simulink model "Get_RE_RhythmCalc_Sig2Mbed_Tcontrol_paper_ver"  (R2013a)
settings: Solver=FixedStepDiscrete  StartTime=0.0  StopTime=65  RelTol=1e-3
values from neighbouring files (symbols this model uses):
  ts = 1/50    (= 0.02)    [arduino_setup.m]
libraries: arduino_io_lib x12, simulink x8
settings Model: Creator=cell  LastModifiedBy=cell
settings OptimizationCC: OptimizeModelRefInitCode=on  LifeSpan=1
settings DebuggingCC: CheckSSInitialOutputMsg=off  InheritedTsInSrcMsg=none  StrictBusMsg=Warning
settings HardwareCC: ProdBitPerInt=16  ProdBitPerPointer=8  ProdIntDivRoundTo=Zero  ProdEndianess=LittleEndian  ProdWordSize=8  ProdHWDeviceType=Atmel->AVR
settings RTWCC: SystemTargetFile=realtime.tlc  GenerateMakefile=off  TemplateMakefile=realtime.tmf  Description=Run on Target Hardware  RTWVerbose=off  ProcessScript=realtime_make_rtw_hook
settings CodeAppCC: IgnoreCustomStorageClasses=off
settings STFCustomTargetCC: TargetLibSuffix=.a  GenerateSampleERTMain=on  CombineOutputUpdateFcns=on  ERTCustomFileBanners=on  SupportContinuousTime=off  SupportNonInlinedSFcns=off  MATLABClassNameForMDSCustomization=Simulink.SoftwareTarget.ERTCustomization  SystemTargetFile=realtime.tlc
settings ERTTargetCC: ParMdlRefBuildCompliant=off  CompOptLevelCompliant=off  ConcurrentExecutionCompliant=off  ERTFirstTimeCompliant=off  ModelStepFunctionPrototypeControlCompliant=off  CPPClassGenCompliant=off  ERTCustomFileTemplate=realtime_file_process.tlc

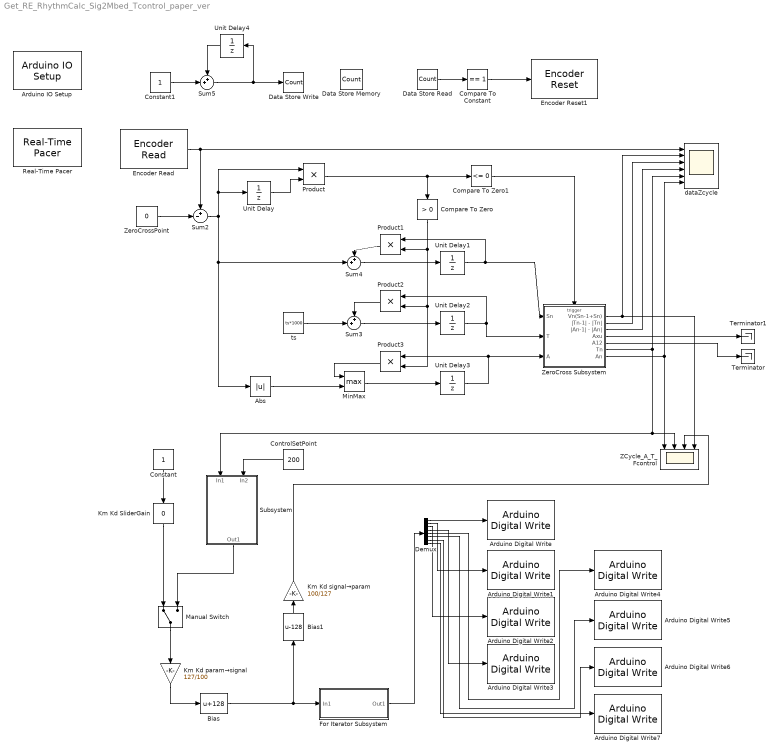
== system Get_RE_RhythmCalc_Sig2Mbed_Tcontrol_paper_ver ==
  Abs : Abs
  Arduino Digital Write : arduino_io_lib/Arduino Digital Write  arduinoVar=Existing workspace arduino variable #1  arduinoPin=6  T=ts
  Arduino Digital Write1 : arduino_io_lib/Arduino Digital Write  arduinoVar=Existing workspace arduino variable #1  arduinoPin=7  T=ts
  Arduino Digital Write2 : arduino_io_lib/Arduino Digital Write  arduinoVar=Existing workspace arduino variable #1  arduinoPin=8  T=ts
  Arduino Digital Write3 : arduino_io_lib/Arduino Digital Write  arduinoVar=Existing workspace arduino variable #1  arduinoPin=9  T=ts
  Arduino Digital Write4 : arduino_io_lib/Arduino Digital Write  arduinoVar=Existing workspace arduino variable #1  arduinoPin=10  T=ts
  Arduino Digital Write5 : arduino_io_lib/Arduino Digital Write  arduinoVar=Existing workspace arduino variable #1  arduinoPin=11  T=ts
  Arduino Digital Write6 : arduino_io_lib/Arduino Digital Write  arduinoVar=Existing workspace arduino variable #1  arduinoPin=12  T=ts
  Arduino Digital Write7 : arduino_io_lib/Arduino Digital Write  arduinoVar=Existing workspace arduino variable #1  arduinoPin=13  T=ts
  Arduino IO Setup : arduino_io_lib/Arduino IO Setup  Priority=3  arduinoVar=Existing workspace arduino variable #1  workspaceVarName=a  comPort=DEMO
  Bias : Bias  Bias=128
  Bias1 : Bias  Bias=-128
  Compare To Constant : simulink/Logic and Bit Operations/Compare To Constant  relop===  const=1  OutDataTypeStr=boolean
  Compare To Zero : simulink/Logic and Bit Operations/Compare To Zero  relop=>  OutDataTypeStr=boolean
  Compare To Zero1 : simulink/Logic and Bit Operations/Compare To Zero  relop=<=  OutDataTypeStr=boolean
  Constant : Constant
  Constant1 : Constant
  ControlSetPoint : Constant  Value=200
  Data Store Memory : DataStoreMemory  DataStoreName=Count  ReadBeforeWriteMsg=warning  WriteAfterWriteMsg=warning  WriteAfterReadMsg=warning
  Data Store Read : DataStoreRead  DataStoreName=Count
  Data Store Write : DataStoreWrite  DataStoreName=Count
  Demux : Demux  Outputs=8
  Encoder Read : arduino_io_lib/Encoder Read  arduinoVar=Existing workspace arduino variable #1  encNum=1  pinA=2  pinB=3  DbDl=0  T=ts
  Encoder Reset1 : arduino_io_lib/Encoder Reset  arduinoVar=Existing workspace arduino variable #1  encNum=1  T=ts
  For Iterator Subsystem : Subsystem  TreatAsAtomicUnit=on  mask{bits=8}
      mask prompts: bits "ビット数"
      mask Display: disp('Integer To Bit\nConvertor')
  Km Kd SliderGain : simulink/Math Operations/Slider Gain  low=-100  gain=0  high=100
  Km Kd param→signal : Gain  Gain=127/100
  Km Kd signal→param : Gain  Gain=100/127
  Manual Switch : ManualSwitch
  MinMax : MinMax  Function=max  Inputs=2  OutDataTypeStr=double
      settings: LockScale=on
  Product{,1..3} (4 alike) : Product
  Real-Time Pacer : arduino_io_lib/Real-Time Pacer  simTimePerRealTime=1
  Subsystem : Subsystem
  Sum2 : Sum  Inputs=+-|
  Sum3 : Sum  Inputs=++|
  Sum4 : Sum  Inputs=++|
  Sum5 : Sum  Inputs=++|
  Terminator : Terminator
  Terminator1 : Terminator
  Unit Delay{,1..4} (5 alike) : UnitDelay  SampleTime=-1
  ZCycle_A_T_Fcontrol : Scope  NumInputPorts=4
      settings: TimeRange=10  YMin=0~0~-50~-250  YMax=175~1400~50~250  SaveName=ZCycle_A_T_Fcontrol
  ZeroCross Subsystem : Subsystem  TreatAsAtomicUnit=on
  ZeroCrossPoint : Constant  Value=0
  dataZcycle : Scope  NumInputPorts=6
      settings: TimeRange=10  YMin=-250~-750~0~0~0~0  YMax=300~2500~400~225~700~500  SaveName=dataZcycle
  ts : Constant  Value=ts*1000
  wires:
  Encoder Read/1 -> dataZcycle/1, Sum2/1
  For Iterator Subsystem/1(Out1) -> Demux/1
  Demux/1 -> Arduino Digital Write/1
  Demux/2 -> Arduino Digital Write1/1
  Demux/3 -> Arduino Digital Write2/1
  Demux/4 -> Arduino Digital Write3/1
  Demux/5 -> Arduino Digital Write4/1
  Demux/6 -> Arduino Digital Write5/1
  Demux/7 -> Arduino Digital Write6/1
  Demux/8 -> Arduino Digital Write7/1
  ZeroCrossPoint/1 -> Sum2/2
  Compare To Zero1/1 -> ZeroCross Subsystem/Trigger
  Product/1 -> Compare To Zero1/1, Compare To Zero/1
  Sum2/1 -> Product/1, Unit Delay/1, Abs/1, Sum4/2
  Product2/1 -> Sum3/1
  Product1/1 -> Sum4/1
  Sum4/1 -> Unit Delay1/1
  ZeroCross Subsystem/3(|An-1| - |An|) -> dataZcycle/4
  Constant1/1 -> Sum5/2
  Sum5/1 -> Unit Delay4/1, Data Store Write/1
  ZeroCross Subsystem/2(|Tn-1| - |Tn|) -> dataZcycle/3
  Product3/1 -> MinMax/1
  Unit Delay4/1 -> Sum5/1
  Data Store Read/1 -> Compare To Constant/1
  Compare To Constant/1 -> Encoder Reset1/1
  ZeroCross Subsystem/6(Tn) -> dataZcycle/5, Subsystem/1(In1), ZCycle_A_T_Fcontrol/2
  ZeroCross Subsystem/7(An) -> dataZcycle/6, ZCycle_A_T_Fcontrol/1
  Constant/1 -> Km Kd SliderGain/1
  Bias/1 -> For Iterator Subsystem/1(In1), Bias1/1
  MinMax/1 -> Unit Delay3/1
  Unit Delay3/1 -> ZeroCross Subsystem/3(A), Product3/1
  Unit Delay2/1 -> ZeroCross Subsystem/2(T), Product2/1
  ts/1 -> Sum3/2
  Unit Delay1/1 -> ZeroCross Subsystem/1(Sn), Product1/1
  ZeroCross Subsystem/4(Axu) -> Terminator1/1
  ZeroCross Subsystem/5(A12) -> Terminator/1
  Subsystem/1(Out1) -> Manual Switch/2
  Unit Delay/1 -> Product/2
  Compare To Zero/1 -> Product3/2, Product2/2, Product1/2
  Sum3/1 -> Unit Delay2/1
  ZeroCross Subsystem/1(Vn(Sn-1+Sn)) -> ZCycle_A_T_Fcontrol/4, dataZcycle/2
  Abs/1 -> MinMax/2
  Manual Switch/1 -> Km Kd param→signal/1
  Km Kd param→signal/1 -> Bias/1
  Km Kd signal→param/1 -> ZCycle_A_T_Fcontrol/3
  Bias1/1 -> Km Kd signal→param/1
  ControlSetPoint/1 -> Subsystem/2(In2)
  Km Kd SliderGain/1 -> Manual Switch/1

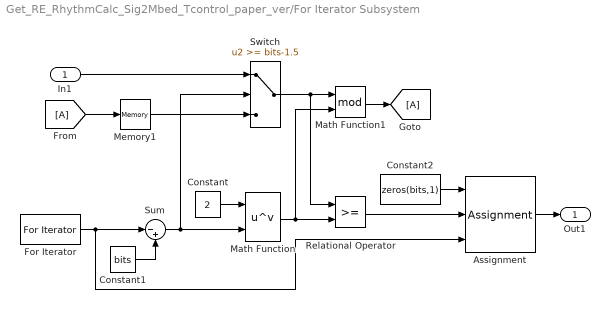
== system Get_RE_RhythmCalc_Sig2Mbed_Tcontrol_paper_ver/For Iterator Subsystem ==
  In1 : Inport
  Assignment : Assignment  IndexOptions=Index vector (port)  Indices=1  OutputSizes=[1 1]
  Constant : Constant  Value=2
  Constant1 : Constant  Value=bits
  Constant2 : Constant  Value=zeros(bits,1)  VectorParams1D=off
  For Iterator : ForIterator  IterationLimit=bits
  Math Function : Math  Operator=pow  SaturateOnIntegerOverflow=on
  Math Function1 : Math  Operator=mod  SaturateOnIntegerOverflow=on
  Memory1 : Memory  InheritSampleTime=on
  Relational Operator : RelationalOperator  OutDataTypeStr=float('double')
  Sum : Sum  Inputs=|-+
  Switch : Switch  Threshold=bits-1.5
  Out1 : Outport
  wires:
  For Iterator/1 -> Sum/1, Assignment/3
  Constant/1 -> Math Function/1
  Sum/1 -> Math Function/2, Switch/2
  Constant1/1 -> Sum/2
  Math Function/1 -> Math Function1/2, Relational Operator/2
  Switch/1 -> Math Function1/1, Relational Operator/1
  In1/1 -> Switch/1
  Memory1/1 -> Switch/3
  Assignment/1 -> Out1/1
  Constant2/1 -> Assignment/1
  Relational Operator/1 -> Assignment/2
  [A] -> Memory1/1
  Math Function1/1 -> [A]

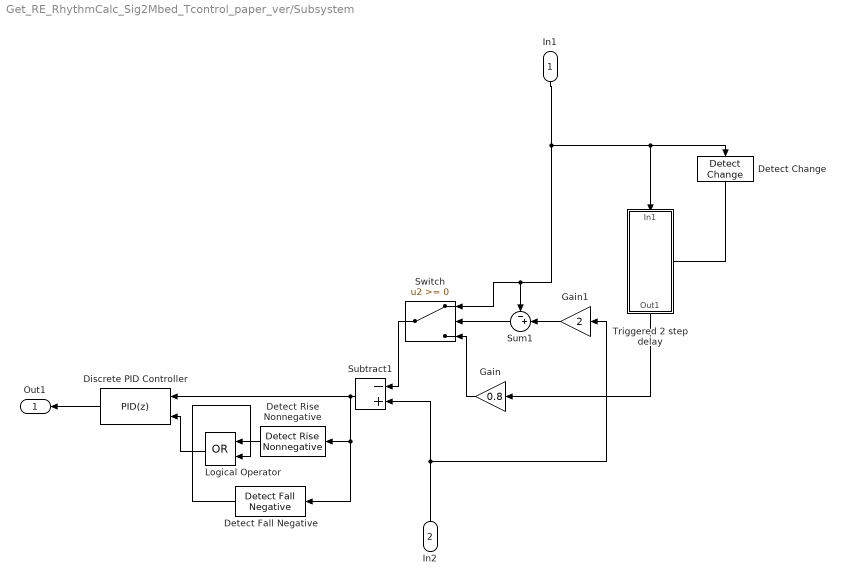
== system Get_RE_RhythmCalc_Sig2Mbed_Tcontrol_paper_ver/Subsystem ==
  In1 : Inport
  In2 : Inport  Port=2
  Detect Change : simulink/Logic and Bit Operations/Detect Change  vinit=0  InputProcessing=Inherited  OutDataTypeStr=boolean
  Detect Fall Negative : simulink/Logic and Bit Operations/Detect Fall Negative  vinit=0  InputProcessing=Inherited  OutDataTypeStr=boolean
  Detect Rise Nonnegative : simulink/Logic and Bit Operations/Detect Rise Nonnegative  vinit=0  InputProcessing=Inherited  OutDataTypeStr=boolean
  Discrete PID Controller : simulink/Continuous/PID Controller  Controller=PID  TimeDomain=Discrete-time  SampleTime=-1  IntegratorMethod=Forward Euler  FilterMethod=Forward Euler  Form=Parallel  P=0.2  I=0.05  D=0  N=100  InitialConditionSource=internal  InitialConditionForIntegrator=0  InitialConditionForFilter=0  ExternalReset=rising  LimitOutput=on  UpperSaturationLimit=50  LowerSaturationLimit=-50  LinearizeAsGain=off  AntiWindupMode=none  Kb=1  TrackingMode=off  Kt=1  PParamMin=[]  PParamMax=[]  IParamMin=[]  IParamMax=[]  DParamMin=[]  DParamMax=[]  NParamMin=[]  NParamMax=[]  KbParamMin=[]  KbParamMax=[]  KtParamMin=[]  KtParamMax=[]  POutMin=[]  POutMax=[]  IOutMin=[]  IOutMax=[]  DOutMin=[]  DOutMax=[]  NOutMin=[]  NOutMax=[]  KbOutMin=[]  KbOutMax=[]  KtOutMin=[]  KtOutMax=[]  IntegratorOutMin=[]  IntegratorOutMax=[]  FilterOutMin=[]  FilterOutMax=[]  SumOutMin=[]  SumOutMax=[]  SumI1OutMin=[]  SumI1OutMax=[]  SumI2OutMin=[]  SumI2OutMax=[]  SumI3OutMin=[]  SumI3OutMax=[]  SumDOutMin=[]  SumDOutMax=[]  SaturationOutMin=[]  SaturationOutMax=[]  IntegratorContinuousStateAttributes=''  IntegratorStateMustResolveToSignalObject=off  IntegratorRTWStateStorageClass=Auto  FilterContinuousStateAttributes=''  FilterStateMustResolveToSignalObject=off  FilterRTWStateStorageClass=Auto
  Gain : Gain  Gain=0.8
  Gain1 : Gain  Gain=2
  Logical Operator : Logic  Operator=OR  AllPortsSameDT=off  OutDataTypeStr=boolean
  Subtract1 : Sum  Inputs=-+
  Sum1 : Sum  Inputs=-+|
  Switch : Switch
  Triggered 2 step delay : Subsystem  TreatAsAtomicUnit=on
  Out1 : Outport
  wires:
  In1/1 -> Sum1/1, Switch/1, Detect Change/1, Triggered 2 step delay/1(In1)
  In2/1 -> Gain1/1, Subtract1/2
  Subtract1/1 -> Detect Fall Negative/1, Detect Rise Nonnegative/1, Discrete PID Controller/1
  Switch/1 -> Subtract1/1
  Gain/1 -> Switch/3
  Gain1/1 -> Sum1/2
  Detect Change/1 -> Triggered 2 step delay/Trigger
  Triggered 2 step delay/1(Out1) -> Gain/1
  Sum1/1 -> Switch/2
  Logical Operator/1 -> Discrete PID Controller/2
  Detect Rise Nonnegative/1 -> Logical Operator/1
  Detect Fall Negative/1 -> Logical Operator/2
  Discrete PID Controller/1 -> Out1/1

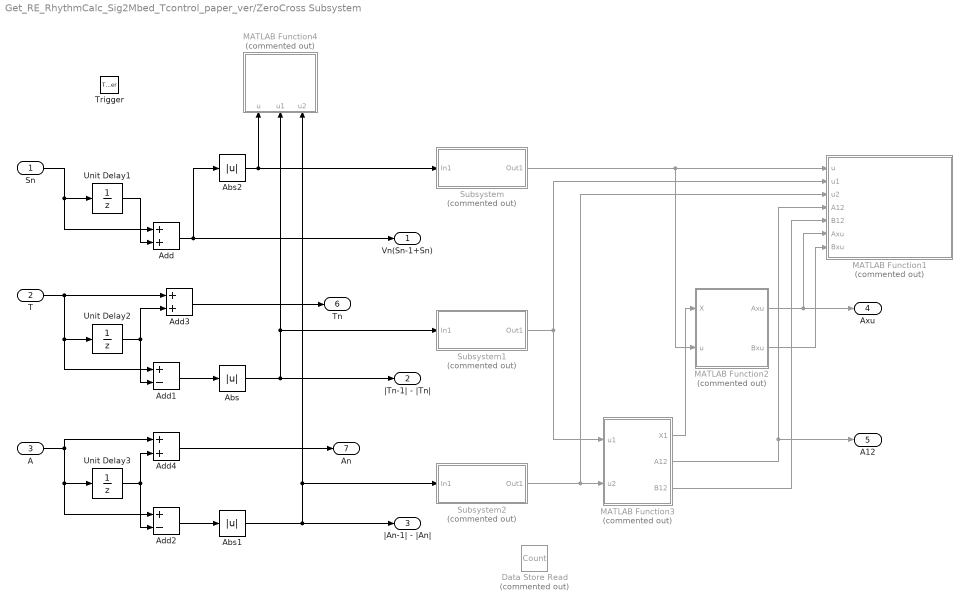
== system Get_RE_RhythmCalc_Sig2Mbed_Tcontrol_paper_ver/ZeroCross Subsystem ==
  Sn : Inport
  T : Inport  Port=2
  A : Inport  Port=3
  Trigger : TriggerPort
  Abs : Abs
  Abs1 : Abs
  Abs2 : Abs
  Add : Sum
  Add1 : Sum  Inputs=+-
  Add2 : Sum  Inputs=+-
  Add3 : Sum
  Add4 : Sum
  Data Store Read : DataStoreRead  Commented=on  DataStoreName=Count
  MATLAB Function1 : MATLAB Function  Commented=on  TreatAsAtomicUnit=on
  MATLAB Function2 : MATLAB Function  Commented=on  TreatAsAtomicUnit=on
  MATLAB Function3 : MATLAB Function  Commented=on  TreatAsAtomicUnit=on
  MATLAB Function4 : MATLAB Function  Commented=on  TreatAsAtomicUnit=on
  Subsystem : Subsystem  Commented=on
  Subsystem1 : Subsystem  Commented=on
  Subsystem2 : Subsystem  Commented=on
  Unit Delay1 : UnitDelay  SampleTime=-1
  Unit Delay2 : UnitDelay  SampleTime=-1
  Unit Delay3 : UnitDelay  SampleTime=-1
  Vn(Sn-1+Sn) : Outport
  |Tn-1| - |Tn| : Outport  Port=2
  |An-1| - |An| : Outport  Port=3
  Axu : Outport  Port=4
  A12 : Outport  Port=5
  Tn : Outport  Port=6
  An : Outport  Port=7
  wires:
  Unit Delay1/1 -> Add/2
  Sn/1 -> Add/1, Unit Delay1/1
  Unit Delay2/1 -> Add1/2, Add3/2
  T/1 -> Add1/1, Unit Delay2/1, Add3/1
  Add1/1 -> Abs/1
  Unit Delay3/1 -> Add4/2, Add2/2
  Add2/1 -> Abs1/1
  Abs1/1 -> |An-1| - |An|/1, MATLAB Function4/3(u2), Subsystem2/1(In1)
  Add/1 -> Abs2/1, Vn(Sn-1+Sn)/1
  Abs/1 -> |Tn-1| - |Tn|/1, Subsystem1/1(In1), MATLAB Function4/2(u1)
  Abs2/1 -> Subsystem/1(In1), MATLAB Function4/1(u)
  Subsystem1/1(Out1) -> MATLAB Function1/2(u1), MATLAB Function3/1(u1)
  Subsystem2/1(Out1) -> MATLAB Function1/3(u2), MATLAB Function3/2(u2)
  MATLAB Function3/1(X1) -> MATLAB Function2/1(X)
  Subsystem/1(Out1) -> MATLAB Function1/1(u), MATLAB Function2/2(u)
  MATLAB Function2/1(Axu) -> Axu/1, MATLAB Function1/6(Axu)
  MATLAB Function2/2(Bxu) -> MATLAB Function1/7(Bxu)
  MATLAB Function3/3(B12) -> MATLAB Function1/5(B12)
  MATLAB Function3/2(A12) -> MATLAB Function1/4(A12), A12/1
  Add3/1 -> Tn/1
  A/1 -> Unit Delay3/1, Add2/1, Add4/1
  Add4/1 -> An/1

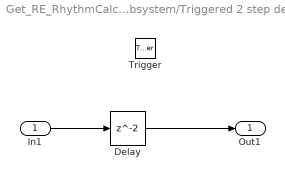
== system Get_RE_RhythmCalc_Sig2Mbed_Tcontrol_paper_ver/Subsystem/Triggered 2 step delay ==
  In1 : Inport
  Trigger : TriggerPort
  Delay : Delay
  Out1 : Outport
  wires:
  In1/1 -> Delay/1
  Delay/1 -> Out1/1

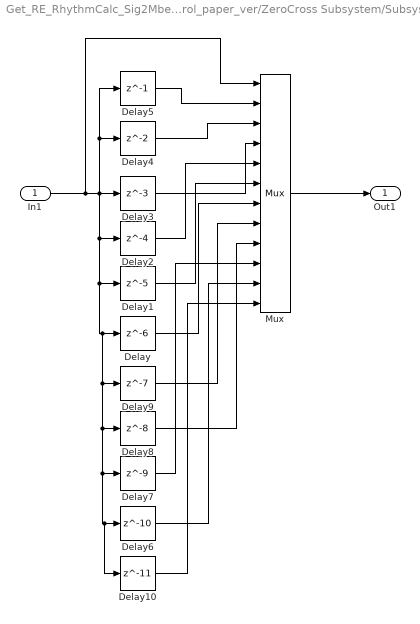
== system Get_RE_RhythmCalc_Sig2Mbed_Tcontrol_paper_ver/ZeroCross Subsystem/Subsystem ==
  In1 : Inport
  Delay : Delay  DelayLength=6
  Delay1 : Delay  DelayLength=5
  Delay10 : Delay  DelayLength=11
  Delay2 : Delay  DelayLength=4
  Delay3 : Delay  DelayLength=3
  Delay4 : Delay
  Delay5 : Delay  DelayLength=1
  Delay6 : Delay  DelayLength=10
  Delay7 : Delay  DelayLength=9
  Delay8 : Delay  DelayLength=8
  Delay9 : Delay  DelayLength=7
  Mux : Mux  Inputs=12
  Out1 : Outport
  wires:
  In1/1 -> Delay5/1, Delay4/1, Delay10/1, Delay6/1, Delay7/1, Delay8/1, Delay9/1, Delay/1, Delay1/1, Delay2/1, Delay3/1, Mux/1
  Delay5/1 -> Mux/2
  Delay4/1 -> Mux/3
  Delay3/1 -> Mux/4
  Delay2/1 -> Mux/5
  Delay1/1 -> Mux/6
  Delay/1 -> Mux/7
  Mux/1 -> Out1/1
  Delay9/1 -> Mux/8
  Delay8/1 -> Mux/9
  Delay7/1 -> Mux/10
  Delay6/1 -> Mux/11
  Delay10/1 -> Mux/12

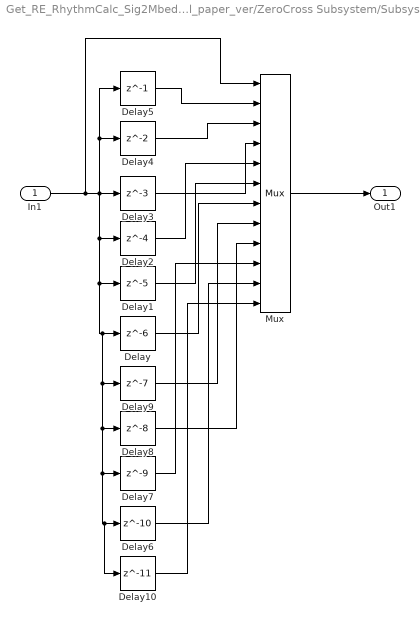
== system Get_RE_RhythmCalc_Sig2Mbed_Tcontrol_paper_ver/ZeroCross Subsystem/Subsystem1 ==
  In1 : Inport
  Delay : Delay  DelayLength=6
  Delay1 : Delay  DelayLength=5
  Delay10 : Delay  DelayLength=11
  Delay2 : Delay  DelayLength=4
  Delay3 : Delay  DelayLength=3
  Delay4 : Delay
  Delay5 : Delay  DelayLength=1
  Delay6 : Delay  DelayLength=10
  Delay7 : Delay  DelayLength=9
  Delay8 : Delay  DelayLength=8
  Delay9 : Delay  DelayLength=7
  Mux : Mux  Inputs=12
  Out1 : Outport
  wires:
  Delay10/1 -> Mux/12
  Delay6/1 -> Mux/11
  Delay7/1 -> Mux/10
  Delay8/1 -> Mux/9
  Delay9/1 -> Mux/8
  Mux/1 -> Out1/1
  Delay/1 -> Mux/7
  Delay1/1 -> Mux/6
  Delay2/1 -> Mux/5
  Delay3/1 -> Mux/4
  Delay4/1 -> Mux/3
  Delay5/1 -> Mux/2
  In1/1 -> Mux/1, Delay3/1, Delay2/1, Delay1/1, Delay/1, Delay9/1, Delay8/1, Delay7/1, Delay6/1, Delay10/1, Delay4/1, Delay5/1

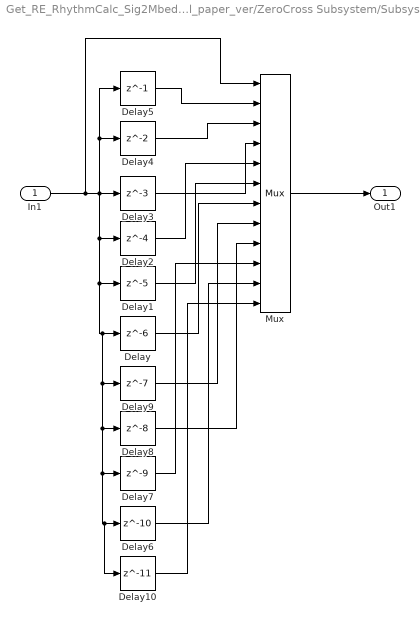
== system Get_RE_RhythmCalc_Sig2Mbed_Tcontrol_paper_ver/ZeroCross Subsystem/Subsystem2 ==
  In1 : Inport
  Delay : Delay  DelayLength=6
  Delay1 : Delay  DelayLength=5
  Delay10 : Delay  DelayLength=11
  Delay2 : Delay  DelayLength=4
  Delay3 : Delay  DelayLength=3
  Delay4 : Delay
  Delay5 : Delay  DelayLength=1
  Delay6 : Delay  DelayLength=10
  Delay7 : Delay  DelayLength=9
  Delay8 : Delay  DelayLength=8
  Delay9 : Delay  DelayLength=7
  Mux : Mux  Inputs=12
  Out1 : Outport
  wires:
  In1/1 -> Delay5/1, Delay4/1, Delay10/1, Delay6/1, Delay7/1, Delay8/1, Delay9/1, Delay/1, Delay1/1, Delay2/1, Delay3/1, Mux/1
  Delay5/1 -> Mux/2
  Delay4/1 -> Mux/3
  Delay3/1 -> Mux/4
  Delay2/1 -> Mux/5
  Delay1/1 -> Mux/6
  Delay/1 -> Mux/7
  Mux/1 -> Out1/1
  Delay9/1 -> Mux/8
  Delay8/1 -> Mux/9
  Delay7/1 -> Mux/10
  Delay6/1 -> Mux/11
  Delay10/1 -> Mux/12

== matlab function Get_RE_RhythmCalc_Sig2Mbed_Tcontrol_paper_ver/ZeroCross Subsystem/MATLAB Function2 ==
  data: X input; u input; Axu output; Bxu output
function [ Axu , Bxu]  = ols_method2( X, u )
%#codegen

% coder.extrinsic('polyfit')
    
% if length(u1) == 7
%     [au12 , bu12]= polyfit(u1 , u2 , 1);
% end

% if Count ==1
%     Sx = sum(u1(1:end-1));
%     Sy = sum(u2(1:end-1));
%     Sxx = sum(u1(1:end-1) .* u1(1:end-1));
%     Sxy = sum( u1(1:end-1) .* u2(1:end-1));
% end

n = length(u);

Sx = sum(X);
Su = sum(u);
Sxx = sum(X .* X);
Sxu = sum(u .* X);

Axu = ( n*Sxu - Sx*Su ) / ( n*Sxx- Sx^2 );

% k1 =  1 / sqrt(1+Axu^2);    k2 = Axu / sqrt(1+Axu^2);
Bxu = ( Sxx * Su - Sxu * Sx ) / ( n*Sxx- Sx^2 );

%     pxv =  polyfit(X1, u);
 
%     Vmin =  polyval( pxv, min(X1) ) ;
%     Vmax =  polyva( pxv, max(X1) ) ;
% 
%     Rotate_inv = [ cos(-theta) sin(-theta); -sin(-theta) cos(-theta)];      % 逆回転行列
%     m1 =Rotate_inv(1,1);    m2 = Rotate_inv(1,2);
%     u1min = m1 * X1min ; %dT
%     u1max = m1 * X1min ; %dT
%     u2min = n1 * X1min ; %dA
%     u2max = n1 * X1min ; %dA
    
%     plot3( u ,u1,u2-buv, 'o','MarkerSize',2);
%     hold on
%         plot3( [0,600*k1]  , [0,600*k2] , [0,0] ,'r' );
%         plot3( [u1min u1max]  , [u2min u2max] , [Vmin Vmax] ,'r' ,'LineWidth',3 );
%         plot3( [u1max u1max] , [u2max u2max] , [0 Vmax] ,'--r' );
%     hold off

% end

== matlab function Get_RE_RhythmCalc_Sig2Mbed_Tcontrol_paper_ver/ZeroCross Subsystem/MATLAB Function4 ==
  data: u input; u1 input; u2 input
function  rhythmPlot( u, u1, u2  )
%#codegen

hold on
plot3( u1,u2, u,  'o','MarkerSize',2);
grid on
axis square
view(-30,25);
xlim([0 600]);            ylim([0 600]);          zlim([0 5000]);
xlabel('dT');    ylabel('dA’');

== matlab function Get_RE_RhythmCalc_Sig2Mbed_Tcontrol_paper_ver/ZeroCross Subsystem/MATLAB Function1 ==
  data: u input; u1 input; u2 input; A12 input; B12 input; Axu input; Bxu input
function  rhythmPlot_regress( u, u1, u2 , A12, B12 , Axu , Bxu )
%#codegen

plot3( u1,u2, u,  'o','MarkerSize',2);
k1 =  1 / sqrt(1+A12^2);    k2 = A12 / sqrt(1+A12^2);
X1max= max( k1*u1 + k2*(u2-B12) );
hold on
plot3( 500*[0 k1] , 500*[0 k2] + B12, [0 0], 'r');
plot3( [0 X1max*k1] ,[0 X1max*k2]+B12 ,[0 Axu*X1max]+Bxu  ,'r' ,'LineWidth',3 );
hold off
grid on
axis square
view(-30,25);
xlim([0 600]);            ylim([0 600]);          zlim([0 5000]);
xlabel('dT');    ylabel('dA');

== matlab function Get_RE_RhythmCalc_Sig2Mbed_Tcontrol_paper_ver/ZeroCross Subsystem/MATLAB Function3 ==
  data: u1 input; u2 input; X1 output; A12 output; B12 output
% function X1   = ols_method1( Sx, Sy, Sxx, Sxy, u1, u2 , Count)
function [ X1 , A12 , B12 ]  = ols_method1( u1, u2 )
%#codegen

% coder.extrinsic('polyfit')
    
% if length(u1) == 7
%     [au12 , bu12]= polyfit(u1 , u2 , 1);
% end

% if Count ==1
%     Sx = sum(u1(1:end-1));
%     Sy = sum(u2(1:end-1));
%     Sxx = sum(u1(1:end-1) .* u1(1:end-1));
%     Sxy = sum( u1(1:end-1) .* u2(1:end-1));
% end

n = length(u1);

S1 = sum(u1);
S2 = sum(u2);
S11 = sum(u1 .* u1);
S12 = sum(u1 .* u2);

A12 = ( n*S12 - S1*S2 ) / ( n*S11- S1^2 );

k1 =  1 / sqrt(1+A12^2);    k2 = A12 / sqrt(1+A12^2);
B12 = ( S11 * S2 - S12 * S1 ) / ( n*S11- S1^2 );
X1 = k1 * u1 + k2 * (u2 - B12);

%     pxv =  polyfit(X1, u);
 
%     Vmin =  polyval( pxv, min(X1) ) ;
%     Vmax =  polyva( pxv, max(X1) ) ;
% 
%     Rotate_inv = [ cos(-theta) sin(-theta); -sin(-theta) cos(-theta)];      % 逆回転行列
%     m1 =Rotate_inv(1,1);    m2 = Rotate_inv(1,2);
%     u1min = m1 * X1min ; %dT
%     u1max = m1 * X1min ; %dT
%     u2min = n1 * X1min ; %dA
%     u2max = n1 * X1min ; %dA
    
%     plot3( u ,u1,u2-buv, 'o','MarkerSize',2);
%     hold on
%         plot3( [0,600*k1]  , [0,600*k2] , [0,0] ,'r' );
%         plot3( [u1min u1max]  , [u2min u2max] , [Vmin Vmax] ,'r' ,'LineWidth',3 );
%         plot3( [u1max u1max] , [u2max u2max] , [0 Vmax] ,'--r' );
%     hold off

% end
